simulink model "sTest_SingleTone_JG"  (R2026a)
settings: Solver=VariableStepAuto  StopTime=0.0001
undefined symbols (not defined in the file or in its folder): Fs, PhaseInc, Ts
libraries: targetingLib x2, dsphdlsigops2 x1
settings Model: Creator=jgovinda  LastModifiedBy=jgovinda

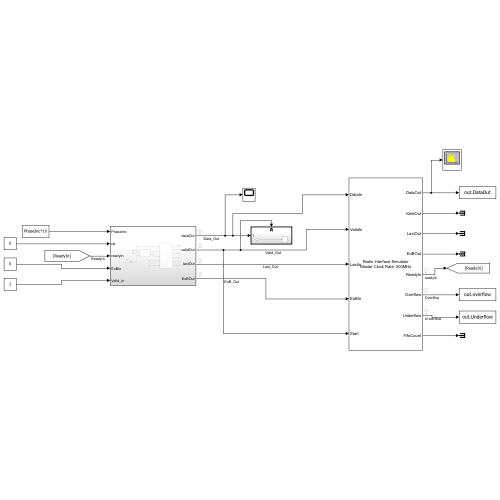
[thumbnail: Simulink's stored preview of the top-level diagram]
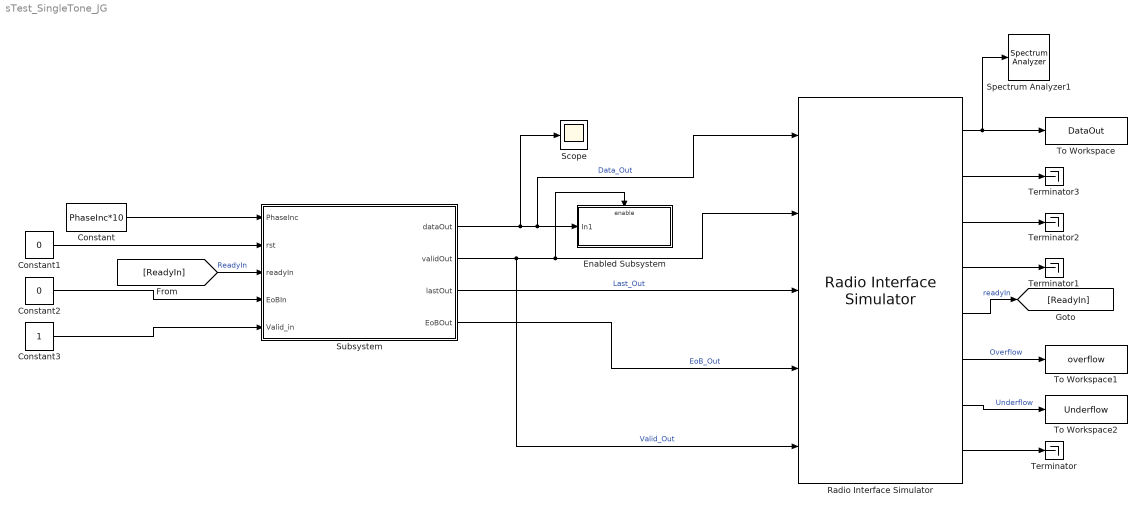
== system sTest_SingleTone_JG ==
  Constant : Constant  Value=PhaseInc*10  OutDataTypeStr=uint16  SampleTime=Ts
  Constant1 : Constant  Value=0  OutDataTypeStr=boolean  SampleTime=Ts
  Constant2 : Constant  Value=0  OutDataTypeStr=boolean  SampleTime=Ts
  Constant3 : Constant  OutDataTypeStr=boolean  SampleTime=Ts
  Enabled Subsystem : Subsystem  TreatAsAtomicUnit=on
  Radio Interface Simulator : targetingLib/Radio Interface Simulator  Device=X310  TXRX=TX  ClockSource=Radio  SampleRate=Fs/2  DUTClockRate=61.44e6  InputDataSource=[ 1, 2, 3 ]  ShowOutputStream=on  SimulateUsing=Interpreted execution  ClockUncertainty=off  Uncertainty=0  Jitter=0
  Scope : Scope
      settings: ActiveDisplayYMinimum=-1.25  ActiveDisplayYMaximum=1.25
  Spectrum Analyzer1 : SpectrumAnalyzer  WindowPosition=[588.000000,199.000000,800.000000,500.000000,]  ScopeFrameLocation=window  WindowInvariantSamplesPerUpdate=on  YLimits=[-55.6845 31.1898]
  Subsystem : Subsystem
  Terminator{,1..3} (4 alike) : Terminator
  To Workspace : ToWorkspace  VariableName=DataOut  SaveFormat=Timeseries  SampleTime=-1
  To Workspace1 : ToWorkspace  VariableName=overflow  SaveFormat=Timeseries  SampleTime=-1
  To Workspace2 : ToWorkspace  VariableName=Underflow  SaveFormat=Timeseries  SampleTime=-1
  wires:
  Subsystem/1(dataOut) -> Scope/1, Enabled Subsystem/1(In1), Radio Interface Simulator/1  "Data_Out"
  Constant/1 -> Subsystem/1(PhaseInc)
  Constant1/1 -> Subsystem/2(rst)
  Constant2/1 -> Subsystem/4(EoBIn)
  Constant3/1 -> Subsystem/5(Valid_in)
  Subsystem/2(validOut) -> Radio Interface Simulator/5, Enabled Subsystem/Enable, Radio Interface Simulator/2  "Valid_Out"
  Subsystem/3(lastOut) -> Radio Interface Simulator/3  "Last_Out"
  Subsystem/4(EoBOut) -> Radio Interface Simulator/4  "EoB_Out"
  [ReadyIn] -> Subsystem/3(readyIn)  "ReadyIn"
  Radio Interface Simulator/8 -> Terminator/1
  Radio Interface Simulator/4 -> Terminator1/1
  Radio Interface Simulator/3 -> Terminator2/1
  Radio Interface Simulator/2 -> Terminator3/1
  Radio Interface Simulator/1 -> Spectrum Analyzer1/1, To Workspace/1
  Radio Interface Simulator/6 -> To Workspace1/1  "Overflow"
  Radio Interface Simulator/7 -> To Workspace2/1  "Underflow"
  Radio Interface Simulator/5 -> [ReadyIn]  "readyIn"

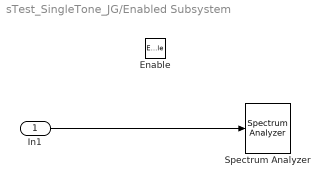
== system sTest_SingleTone_JG/Enabled Subsystem ==
  In1 : Inport
  Enable : EnablePort
  Spectrum Analyzer : SpectrumAnalyzer  WindowPosition=[-9.000000,197.000000,800.000000,500.000000,]  ScopeFrameLocation=window  WindowInvariantSamplesPerUpdate=on  YLimits=[-41.0043 36.876]
  wires:
  In1/1 -> Spectrum Analyzer/1

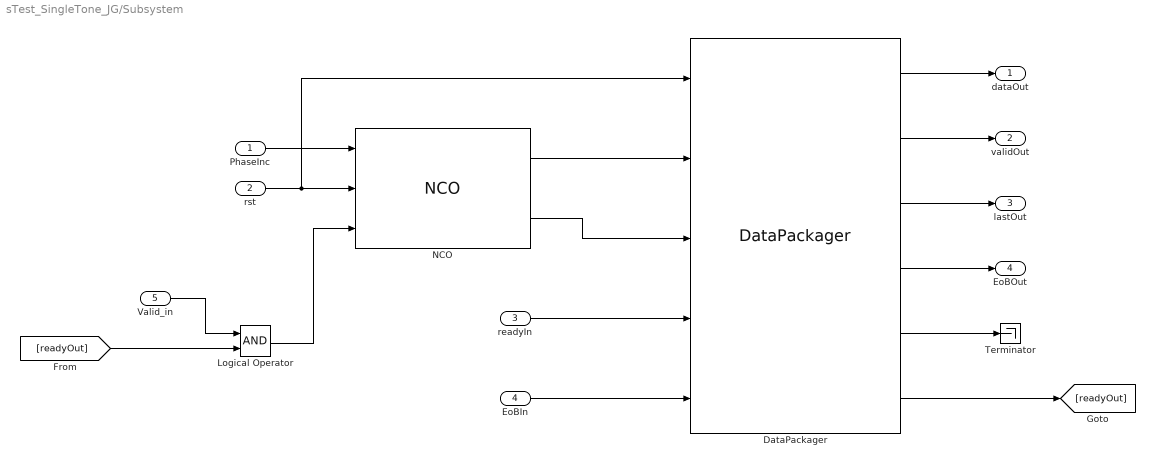
== system sTest_SingleTone_JG/Subsystem ==
  PhaseInc : Inport
  rst : Inport  Port=2
  readyIn : Inport  Port=3
  EoBIn : Inport  Port=4
  Valid_in : Inport  Port=5
  DataPackager : targetingLib/DataPackager  SystemSampleTime=-1  VariantActivationTime=update diagram  EmptyChoice=off  PassThrough=off  PassThroughVariantControl=(default)  EmptyChoiceVariantControl=(default)  AllowFlexibleInterface=on  Latency=0  AutoFrameSizeCalculation=off
  Logical Operator : Logic  AllPortsSameDT=off  OutDataTypeStr=boolean
  NCO : dsphdlsigops2/NCO  PhaseIncrementSource=Input port  PhaseIncrement=100  Frequency=510  FreqResolution=0.05  SamplingFreq=4000  PhaseOffsetSource=Property  PhaseOffset=0  PhaseOffsetR=pi/3  DitherSource=Property  NumDitherBits=4  SamplesPerFrame=1  LUTCompress=off  ResetAction=on  Waveform=Complex exponential  PhasePort=off  SimulateUsing=Code generation  AccumulatorWL=16  PhaseQuantization=on  NumQuantizerAccumulatorBits=12  OutputDataType=Binary point scaling  OutputWL=16  OutputFL=14
      settings: LibrarySourceBlock=dsphdlsrcs2/NCO
  Terminator : Terminator
  dataOut : Outport
  validOut : Outport  Port=2
  lastOut : Outport  Port=3
  EoBOut : Outport  Port=4
  wires:
  NCO/1 -> DataPackager/2
  NCO/2 -> DataPackager/3
  PhaseInc/1 -> NCO/1
  rst/1 -> DataPackager/1, NCO/2
  readyIn/1 -> DataPackager/4
  EoBIn/1 -> DataPackager/5
  DataPackager/1 -> dataOut/1
  DataPackager/2 -> validOut/1
  DataPackager/3 -> lastOut/1
  DataPackager/4 -> EoBOut/1
  DataPackager/5 -> Terminator/1
  Logical Operator/1 -> NCO/3
  Valid_in/1 -> Logical Operator/1
  [readyOut] -> Logical Operator/2
  DataPackager/6 -> [readyOut]
